simulink subsystem "multirotor_angles_sim"  (R2023b)
settings: Solver=VariableStepAuto  StartTime=0.0  StopTime=10.0  RelTol=1e-3
settings Model: Creator=minu_  LastModifiedBy=minu_

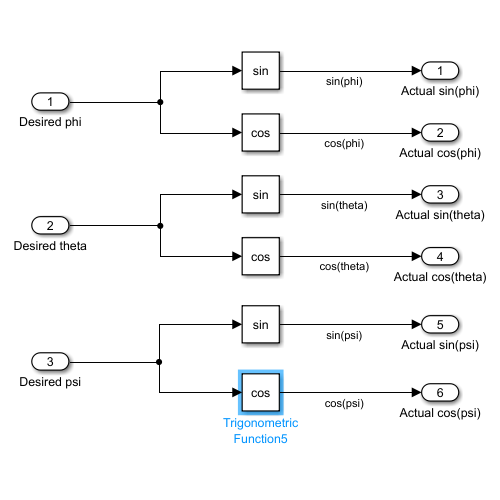
[thumbnail: Simulink's stored preview of the top-level diagram]
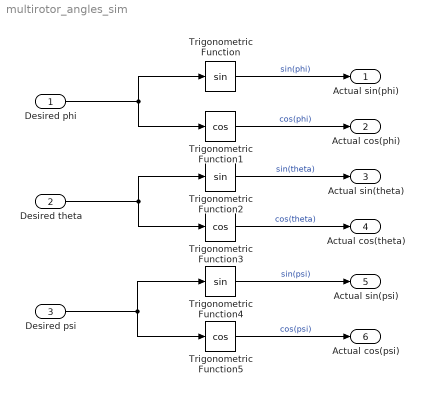
== system multirotor_angles_sim ==
  Desired phi : Inport
  Desired theta : Inport  Port=2
  Desired psi : Inport  Port=3
  Trigonometric Function : Trigonometry
  Trigonometric Function1 : Trigonometry  Operator=cos
  Trigonometric Function2 : Trigonometry
  Trigonometric Function3 : Trigonometry  Operator=cos
  Trigonometric Function4 : Trigonometry
  Trigonometric Function5 : Trigonometry  Operator=cos
  Actual sin(phi) : Outport
  Actual cos(phi) : Outport  Port=2
  Actual sin(theta) : Outport  Port=3
  Actual cos(theta) : Outport  Port=4
  Actual sin(psi) : Outport  Port=5
  Actual cos(psi) : Outport  Port=6
  wires:
  Trigonometric Function1/1 -> Actual cos(phi)/1  "cos(phi)"
  Desired theta/1 -> Trigonometric Function3/1, Trigonometric Function2/1
  Trigonometric Function3/1 -> Actual cos(theta)/1  "cos(theta)"
  Desired psi/1 -> Trigonometric Function4/1, Trigonometric Function5/1
  Trigonometric Function/1 -> Actual sin(phi)/1  "sin(phi)"
  Trigonometric Function2/1 -> Actual sin(theta)/1  "sin(theta)"
  Trigonometric Function5/1 -> Actual cos(psi)/1  "cos(psi)"
  Desired phi/1 -> Trigonometric Function1/1, Trigonometric Function/1
  Trigonometric Function4/1 -> Actual sin(psi)/1  "sin(psi)"
